simulink model "tut6"  (R2024a)
settings: Solver=VariableStepAuto  StartTime=0.0  StopTime=10.0  RelTol=1e-3
settings Model: Creator=User  LastModifiedBy=User

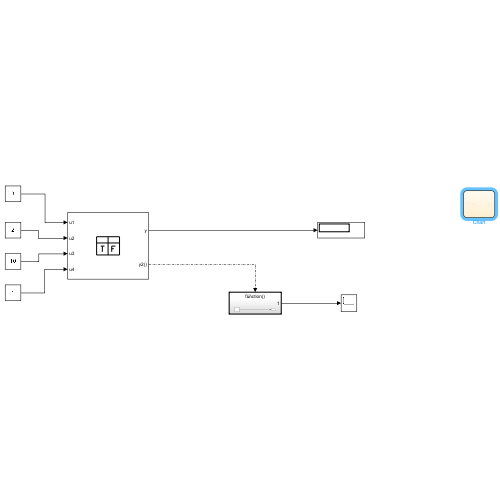
[thumbnail: Simulink's stored preview of the top-level diagram]
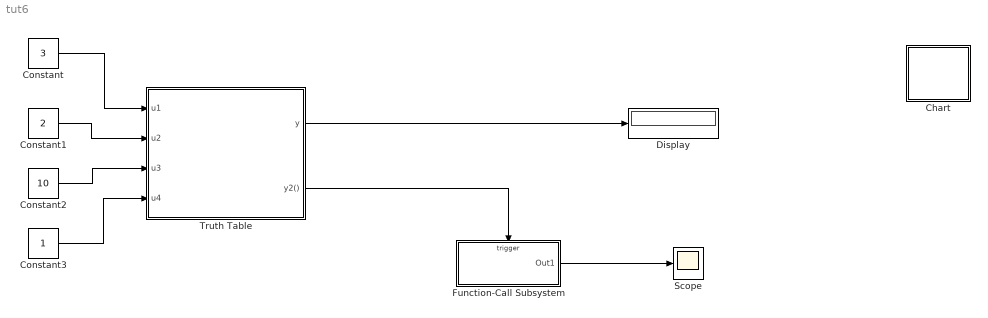
== system tut6 ==
  Chart : Stateflow chart  TreatAsAtomicUnit=on
  Constant : Constant  Value=3
  Constant1 : Constant  Value=2
  Constant2 : Constant  Value=10
  Constant3 : Constant
  Display : Display
  Function-Call Subsystem : Subsystem  TreatAsAtomicUnit=on
  Scope : Scope
  Truth Table : Truth Table  TreatAsAtomicUnit=on
  wires:
  Truth Table/1(y) -> Display/1
  Truth Table/2(y2()) -> Function-Call Subsystem/Trigger
  Function-Call Subsystem/1(Out1) -> Scope/1
  Constant1/1 -> Truth Table/2(u2)
  Constant2/1 -> Truth Table/3(u3)
  Constant3/1 -> Truth Table/4(u4)
  Constant/1 -> Truth Table/1(u1)

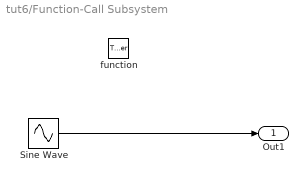
== system tut6/Function-Call Subsystem ==
  function : TriggerPort  TriggerType=function-call  VariantControl=(inherit)
  Sine Wave : Sin
  Out1 : Outport
  wires:
  Sine Wave/1 -> Out1/1

== matlab function tut6/Truth Table ==
  data: u1 input; y output; u2 input double; u3 input double; u4 input double
  events: y2 output FUNCTION_CALL_EVENT
function y = fcn(u1, u2, u3, u4)

aVarTruthTableCondition_1 = false;
aVarTruthTableCondition_2 = false;
aVarTruthTableCondition_3 = false;
aVarTruthTableCondition_4 = false;
aVarTruthTableCondition_5 = false;
aVarTruthTableCondition_6 = false;


% Example condition 1

aVarTruthTableCondition_1 = logical(u1 > u2);

% Example condition 2

aVarTruthTableCondition_2 = logical(u1>u3);

% Condition #3
aVarTruthTableCondition_3 = logical(u1>u4);

% Condition #4
aVarTruthTableCondition_4 = logical(u2>u3);

% Condition #5
aVarTruthTableCondition_5 = logical(u2>u4);

% Condition #6
aVarTruthTableCondition_6 = logical(u3>u4);

if (aVarTruthTableCondition_1 && aVarTruthTableCondition_2 && aVarTruthTableCondition_3)
    aFcnTruthTableAction_1();
elseif (~aVarTruthTableCondition_1 && aVarTruthTableCondition_4 && aVarTruthTableCondition_5)
    aFcnTruthTableAction_2();
elseif (~aVarTruthTableCondition_2 && ~aVarTruthTableCondition_4 && aVarTruthTableCondition_6)
    aFcnTruthTableAction_3();
elseif (~aVarTruthTableCondition_3 && ~aVarTruthTableCondition_5 && ~aVarTruthTableCondition_6)
    aFcnTruthTableAction_4();
else % Default
    aFcnTruthTableAction_1();
end

function aFcnTruthTableAction_1()

% Example action 1 called from D1 & D2 column in condition table

y = u1;

function aFcnTruthTableAction_2()

% Example action 2 called from D3 column in condition table

y = u2;

function aFcnTruthTableAction_3()



y=u3;
y2();

function aFcnTruthTableAction_4()



y=u4;

== stateflow chart tut6/Chart ==
  state On
  state Off
  state y=f(u) [function]
    (default) -> (junction 7)
    (junction 7) -> (junction 11) [order 1] : [u>5]
    (junction 11) -> (junction 13) : {x=15;}
    (junction 7) -> (junction 15) [order 2]
  (default) -> On
  On -> Off
  Off -> On
  data: u function_input; y function_output
